simulink model "Lab2"  (R2021a)
settings: Solver=VariableStepAuto  StartTime=0.0  StopTime=60  RelTol=1e-3
values from neighbouring files (symbols this model uses):
  Hcic = tf((6.392-5.81)/11, [5.81, 1])    [Laboratory2.m]
  Hqc = tf((6.041-5.81)/11, [5.52, 1])    [Laboratory2.m]
  Hregulator = minreal(Hregulatorqc)    [Laboratory2.m]
  V = 100    [Laboratory2.m]
undefined symbols (not defined in the file or in its folder): c0, ci, Edr, k0, q
settings Model: Creator=Automatica  LastModifiedBy=Automatica

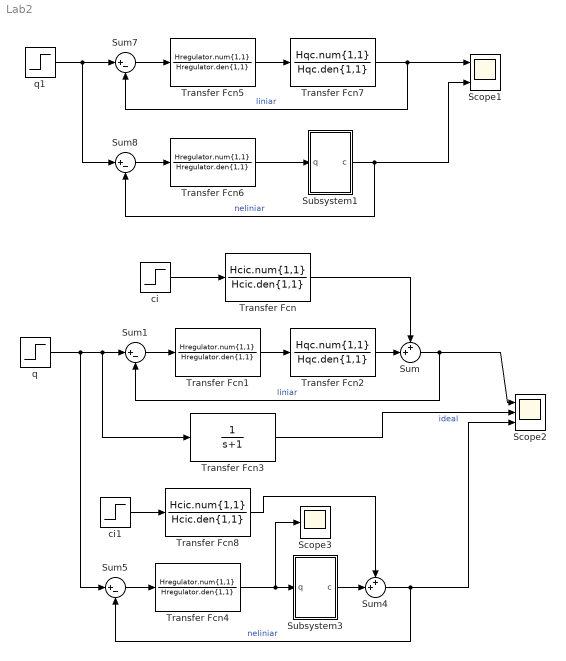
== system Lab2 ==
  Scope1 : Scope  NumInputPorts=2
  Scope2 : Scope  NumInputPorts=3
  Scope3 : Scope
  Subsystem1 : Subsystem
  Subsystem3 : Subsystem
  Sum : Sum  Inputs=++|
  Sum{1,5,7..8} (4 alike) : Sum  Inputs=|+-
  Sum4 : Sum  Inputs=++|
  Transfer Fcn : TransferFcn  Numerator=Hcic.num{1,1}  Denominator=Hcic.den{1,1}
  Transfer Fcn{1,4..6} (4 alike) : TransferFcn  Numerator=Hregulator.num{1,1}  Denominator=Hregulator.den{1,1}
  Transfer Fcn2 : TransferFcn  Numerator=Hqc.num{1,1}  Denominator=Hqc.den{1,1}
  Transfer Fcn3 : TransferFcn  Numerator=1  Denominator=[1, 1]
  Transfer Fcn7 : TransferFcn  Numerator=Hqc.num{1,1}  Denominator=Hqc.den{1,1}
  Transfer Fcn8 : TransferFcn  Numerator=Hcic.num{1,1}  Denominator=Hcic.den{1,1}
  ci : Step  Time=30  Before=ci  After=50  SampleTime=0
  ci1 : Step  Time=30  Before=ci  After=50  SampleTime=0
  q : Step  Time=0  After=q  SampleTime=0
  q1 : Step  Time=0  After=q  SampleTime=0
  wires:
  Transfer Fcn1/1 -> Transfer Fcn2/1
  Transfer Fcn2/1 -> Sum/2
  Sum1/1 -> Transfer Fcn1/1
  Sum/1 -> Scope2/1, Sum1/2  "liniar"
  Transfer Fcn4/1 -> Scope3/1, Subsystem3/1(q)
  Sum5/1 -> Transfer Fcn4/1
  ci/1 -> Transfer Fcn/1
  Sum4/1 -> Scope2/3, Sum5/2  "neliniar"
  Transfer Fcn/1 -> Sum/1
  Transfer Fcn6/1 -> Subsystem1/1(q)
  Transfer Fcn5/1 -> Transfer Fcn7/1
  Subsystem1/1(c) -> Scope1/2, Sum8/2  "neliniar"
  Sum8/1 -> Transfer Fcn6/1
  q1/1 -> Sum8/1, Sum7/1
  Sum7/1 -> Transfer Fcn5/1
  Transfer Fcn7/1 -> Sum7/2, Scope1/1  "liniar"
  q/1 -> Transfer Fcn3/1, Sum1/1, Sum5/1
  ci1/1 -> Transfer Fcn8/1
  Subsystem3/1(c) -> Sum4/2
  Transfer Fcn8/1 -> Sum4/1
  Transfer Fcn3/1 -> Scope2/2  "ideal"

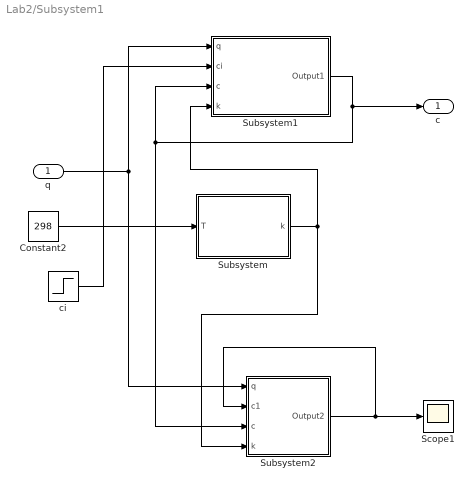
== system Lab2/Subsystem1 ==
  q : Inport
  Constant2 : Constant  Value=298
  Scope1 : Scope
  Subsystem : Subsystem
  Subsystem1 : Subsystem
  Subsystem2 : Subsystem
  ci : Step  Time=0  After=ci  SampleTime=0
  c : Outport
  wires:
  Subsystem/1(k) -> Subsystem2/4(k), Subsystem1/4(k)
  Subsystem2/1(Output2) -> Scope1/1, Subsystem2/2(c1)
  Subsystem1/1(Output1) -> c/1, Subsystem2/3(c), Subsystem1/3(c)
  ci/1 -> Subsystem1/2(ci)
  Constant2/1 -> Subsystem/1(T)
  q/1 -> Subsystem2/1(q), Subsystem1/1(q)

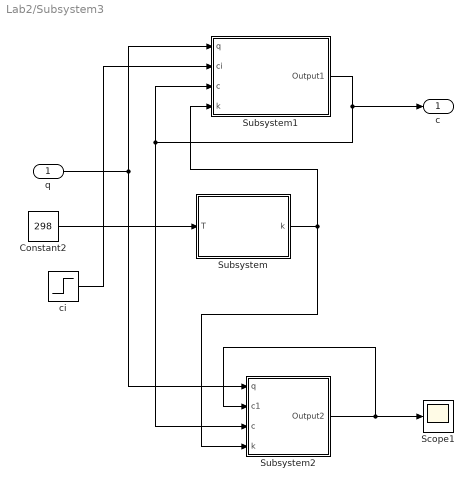
== system Lab2/Subsystem3 ==
  q : Inport
  Constant2 : Constant  Value=298
  Scope1 : Scope
  Subsystem : Subsystem
  Subsystem1 : Subsystem
  Subsystem2 : Subsystem
  ci : Step  Time=0  After=ci  SampleTime=0
  c : Outport
  wires:
  Subsystem/1(k) -> Subsystem2/4(k), Subsystem1/4(k)
  Subsystem2/1(Output2) -> Scope1/1, Subsystem2/2(c1)
  Subsystem1/1(Output1) -> c/1, Subsystem2/3(c), Subsystem1/3(c)
  ci/1 -> Subsystem1/2(ci)
  Constant2/1 -> Subsystem/1(T)
  q/1 -> Subsystem2/1(q), Subsystem1/1(q)

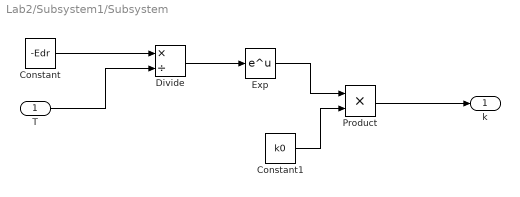
== system Lab2/Subsystem1/Subsystem ==
  T : Inport
  Constant : Constant  Value=-Edr
  Constant1 : Constant  Value=k0
  Divide : Product  Inputs=*/
  Exp : Math  SaturateOnIntegerOverflow=on
  Product : Product
  k : Outport
  wires:
  Exp/1 -> Product/1
  Constant/1 -> Divide/1
  Product/1 -> k/1
  Divide/1 -> Exp/1
  Constant1/1 -> Product/2
  T/1 -> Divide/2

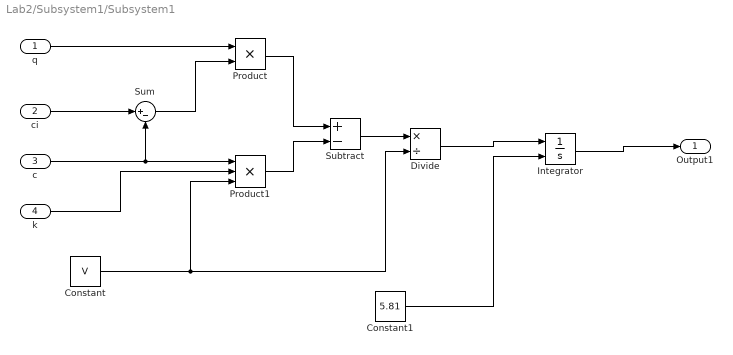
== system Lab2/Subsystem1/Subsystem1 ==
  q : Inport
  ci : Inport  Port=2
  c : Inport  Port=3
  k : Inport  Port=4
  Constant : Constant  Value=V
  Constant1 : Constant  Value=5.81
  Divide : Product  Inputs=*/
  Integrator : Integrator  InitialConditionSource=external  InitialCondition=c0
  Product : Product
  Product1 : Product  Inputs=3
  Subtract : Sum  Inputs=+-
  Sum : Sum  Inputs=|+-
  Output1 : Outport
  wires:
  Product/1 -> Subtract/1
  Integrator/1 -> Output1/1
  Divide/1 -> Integrator/1
  Subtract/1 -> Divide/1
  q/1 -> Product/1
  Constant/1 -> Divide/2, Product1/3
  Sum/1 -> Product/2
  Constant1/1 -> Integrator/2
  c/1 -> Sum/2, Product1/1
  ci/1 -> Sum/1
  k/1 -> Product1/2
  Product1/1 -> Subtract/2

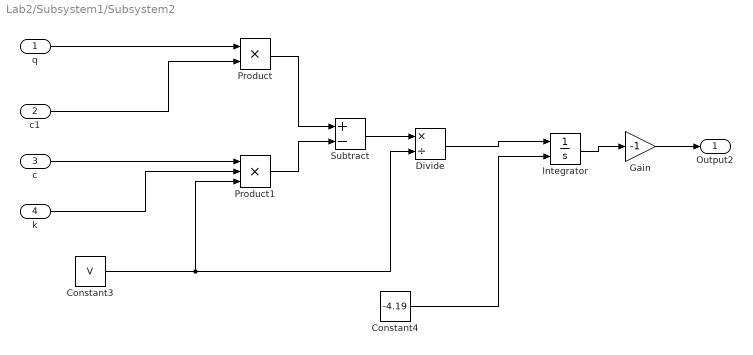
== system Lab2/Subsystem1/Subsystem2 ==
  q : Inport
  c1 : Inport  Port=2
  c : Inport  Port=3
  k : Inport  Port=4
  Constant3 : Constant  Value=V
  Constant4 : Constant  Value=-4.19
  Divide : Product  Inputs=*/
  Gain : Gain  Gain=-1
  Integrator : Integrator  InitialConditionSource=external  InitialCondition=c0
  Product : Product
  Product1 : Product  Inputs=3
  Subtract : Sum  Inputs=+-
  Output2 : Outport
  wires:
  Product/1 -> Subtract/1
  Constant3/1 -> Divide/2, Product1/3
  Product1/1 -> Subtract/2
  c/1 -> Product1/1
  Divide/1 -> Integrator/1
  Subtract/1 -> Divide/1
  q/1 -> Product/1
  k/1 -> Product1/2
  Constant4/1 -> Integrator/2
  c1/1 -> Product/2
  Gain/1 -> Output2/1
  Integrator/1 -> Gain/1

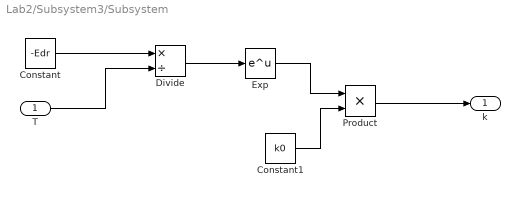
== system Lab2/Subsystem3/Subsystem ==
  T : Inport
  Constant : Constant  Value=-Edr
  Constant1 : Constant  Value=k0
  Divide : Product  Inputs=*/
  Exp : Math  SaturateOnIntegerOverflow=on
  Product : Product
  k : Outport
  wires:
  Exp/1 -> Product/1
  Constant/1 -> Divide/1
  Product/1 -> k/1
  Divide/1 -> Exp/1
  Constant1/1 -> Product/2
  T/1 -> Divide/2

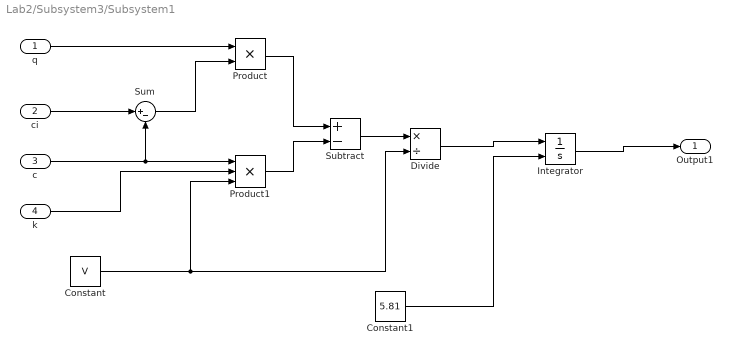
== system Lab2/Subsystem3/Subsystem1 ==
  q : Inport
  ci : Inport  Port=2
  c : Inport  Port=3
  k : Inport  Port=4
  Constant : Constant  Value=V
  Constant1 : Constant  Value=5.81
  Divide : Product  Inputs=*/
  Integrator : Integrator  InitialConditionSource=external  InitialCondition=c0
  Product : Product
  Product1 : Product  Inputs=3
  Subtract : Sum  Inputs=+-
  Sum : Sum  Inputs=|+-
  Output1 : Outport
  wires:
  Product/1 -> Subtract/1
  Integrator/1 -> Output1/1
  Divide/1 -> Integrator/1
  Subtract/1 -> Divide/1
  q/1 -> Product/1
  Constant/1 -> Divide/2, Product1/3
  Sum/1 -> Product/2
  Constant1/1 -> Integrator/2
  c/1 -> Sum/2, Product1/1
  ci/1 -> Sum/1
  k/1 -> Product1/2
  Product1/1 -> Subtract/2

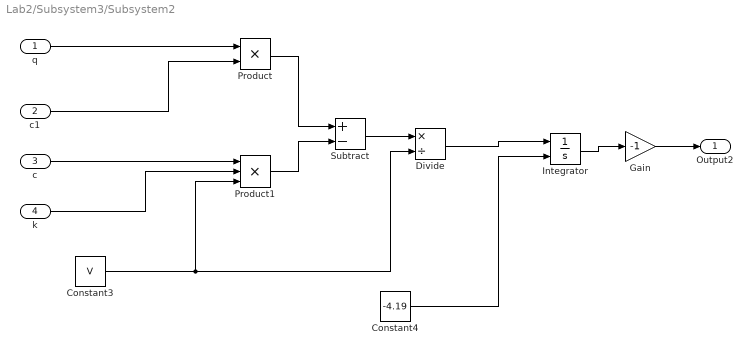
== system Lab2/Subsystem3/Subsystem2 ==
  q : Inport
  c1 : Inport  Port=2
  c : Inport  Port=3
  k : Inport  Port=4
  Constant3 : Constant  Value=V
  Constant4 : Constant  Value=-4.19
  Divide : Product  Inputs=*/
  Gain : Gain  Gain=-1
  Integrator : Integrator  InitialConditionSource=external  InitialCondition=c0
  Product : Product
  Product1 : Product  Inputs=3
  Subtract : Sum  Inputs=+-
  Output2 : Outport
  wires:
  Product/1 -> Subtract/1
  Constant3/1 -> Divide/2, Product1/3
  Product1/1 -> Subtract/2
  c/1 -> Product1/1
  Divide/1 -> Integrator/1
  Subtract/1 -> Divide/1
  q/1 -> Product/1
  k/1 -> Product1/2
  Constant4/1 -> Integrator/2
  c1/1 -> Product/2
  Gain/1 -> Output2/1
  Integrator/1 -> Gain/1
